simulink model "sim_test"  (R2024b)
settings: Solver=VariableStepAuto  StartTime=0.0  StopTime=100  MaxStep=0.001  RelTol=1e-3
values from neighbouring files (symbols this model uses):
  Fmax = 3*m*g    (= 30)    [Test_application.m]
  g = 10    [Test_application.m]
  K = 1    [Test_application.m]
  lover = -m*g    (= -10)    [Test_application.m]
  m = 1    [Test_application.m]
  T = 0.026    [Test_application.m]
settings Model: Creator=Vladimir  LastModifiedBy=Vladimir
settings SFSimCC: UsePrecompiledLibraries=Avoid  SimTargetLang=C++  GPUAcceleration=on  SimDLTargetLibrary=cudnn

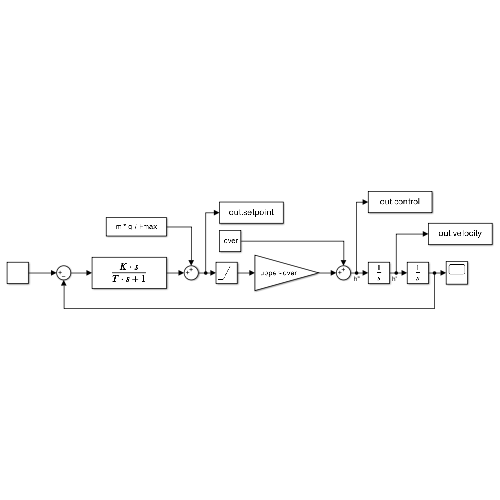
[thumbnail: Simulink's stored preview of the top-level diagram]
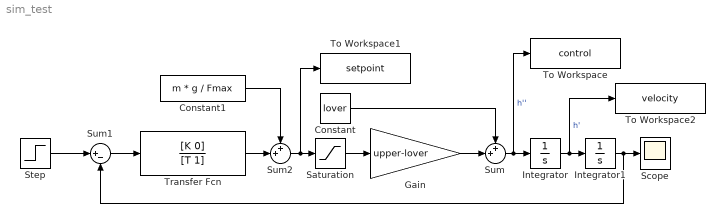
== system sim_test ==
  Constant : Constant  Value=lover
  Constant1 : Constant  Value=m * g / Fmax
  Gain : Gain  Gain=upper-lover
  Integrator : Integrator
  Integrator1 : Integrator
  Saturation : Saturate  UpperLimit=1  LowerLimit=0
  Scope : Scope
  Step : Step  Time=0  SampleTime=0
  Sum : Sum  Inputs=++|
  Sum1 : Sum  Inputs=|+-
  Sum2 : Sum  Inputs=++|
  To Workspace : ToWorkspace  VariableName=control  SampleTime=-1
  To Workspace1 : ToWorkspace  VariableName=setpoint  SampleTime=-1
  To Workspace2 : ToWorkspace  VariableName=velocity  SampleTime=-1
  Transfer Fcn : TransferFcn  Numerator=[K 0]  Denominator=[T 1]
  wires:
  Constant/1 -> Sum/1
  Saturation/1 -> Gain/1
  Gain/1 -> Sum/2
  Sum/1 -> To Workspace/1, Integrator/1  "h''"
  Integrator/1 -> To Workspace2/1, Integrator1/1  "h'"
  Integrator1/1 -> Sum1/2, Scope/1
  Step/1 -> Sum1/1
  Sum2/1 -> To Workspace1/1, Saturation/1
  Constant1/1 -> Sum2/1
  Sum1/1 -> Transfer Fcn/1
  Transfer Fcn/1 -> Sum2/2
